simulink model "Combined_TorqueIncrease"  (Simulink 7.6)
settings: Solver=ode23tb  StartTime=0.0  StopTime=5  RelTol=1e-3
libraries: powerlib x14, powerlib_extras x1
settings Model: Creator=kif  LastModifiedBy=kif

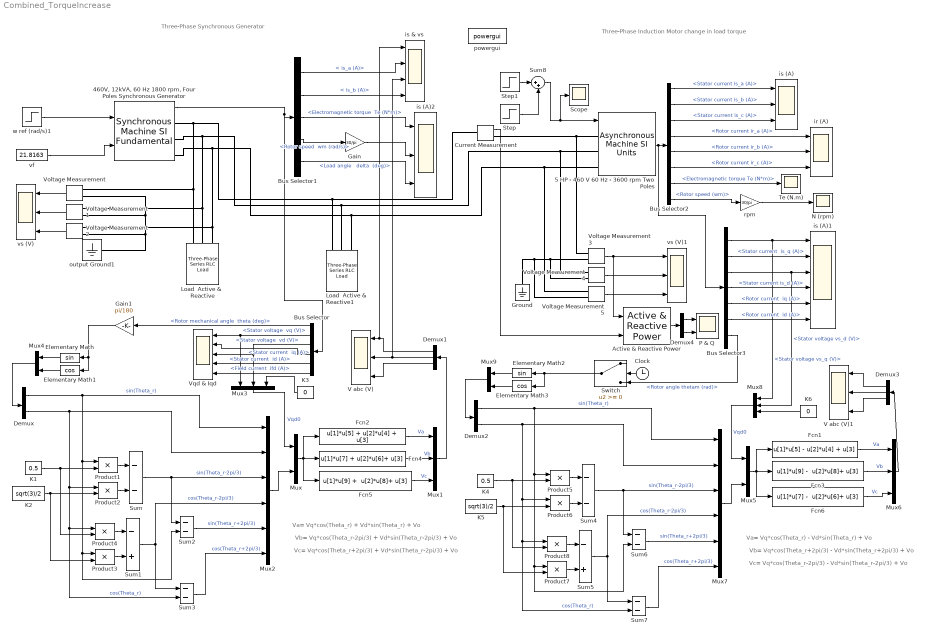
== system Combined_TorqueIncrease ==
  note: Three-Phase Synchronous Generator
  note: Va= Vq*cos(Theta_r) + Vd*sin(Theta_r) + Vo
  note: Vc= Vq*cos(Theta_r+2pi/3) + Vd*sin(Theta_r-2pi/3) + Vo
  note: Vb= Vq*cos(Theta_r-2pi/3) + Vd*sin(Theta_r-2pi/3) + Vo
  note: Three-Phase Induction Motor change in load torque
  note: Va= Vq*cos(Theta_r) - Vd*sin(Theta_r) + Vo
  note: Vc= Vq*cos(Theta_r-2pi/3) - Vd*sin(Theta_r-2pi/3) + Vo
  note: Vb= Vq*cos(Theta_r+2pi/3) - Vd*sin(Theta_r+2pi/3) + Vo
  "460V, 12kVA, 60 Hz 1800 rpm, Four Poles Synchronous Generator" : powerlib/Machines/Synchronous Machine SI Fundamental  DialogController=POWERSYS.PowerSysDialog  SystemSampleTime=-1  PresetModel=No  MechanicalLoad=Speed w  ShowDetailedParameters=on  RotorType=Salient-pole  NominalParameters="[ 11.9e3 460  60  0]"  Stator=[ .26 1.14e-3 13.7e-3 11.0e-3 ]  Field=[ 0.3 2.1e-3 ]  Dampers2=[ 1 2 3 4 5 6 ]  Dampers1=[ 0.0224 1.4e-3 0.02 1e-3 ]  Mechanical=[ 24.9 0 2]  PolePairs=2  InitialConditions=[0 -111.483 0 0 0 -173.297 66.7033 -53.2967 17.88]  SetSaturation=off  Saturation=[46.376,51.647,61.167,66.773,72.147,78.393,86.24,95.347,105.58;644,708.2,816.2,870.87,917.13,962.47,1012,1059.3,1104.5]  DisplayVfd=off  Units=SI fundamental parameters  LoadFlowParameters=[1 -50000 0 0 0]  TsPowergui=0  TsBlock=-1  IterativeModel=Forward Euler
      link override From: GotoTag=tp5344ed80_c545_43ed_8e4c_276f4009b387
      settings: AttributesFormatString=\n
  5 HP - 460 V 60 Hz - 3600 rpm Two Poles : powerlib/Machines/Asynchronous Machine SI Units  DialogController=POWERSYS.PowerSysDialog  SystemSampleTime=-1  PresetModel=No  MechanicalLoad=Torque Tm  ShowDetailedParameters=on  RotorType=Squirrel-cage  ReferenceFrame=Stationary  NominalParameters=[3730 460 60]  Stator=[1.115 0.005974]  Rotor=[1.083 0.005974]  Cage1=[ 0.022 0.226/377]  Cage2=[ 0.022 0.226/377]  Lm=0.2037  Mechanical=[0.02 0.005752 2]  PolePairs=2  InitialConditions="[ 1,0   0,0,0   0,0,0 ]"  Units=SI  LoadFlowParameters=0  SimulateSaturation=off  Saturation=[14.03593122, 27.81365428, 53.79336849, 72.68890987, 97.98006896, 148.6815601, 215.7428561, 302.9841135, 428.7778367 ; 230, 322, 414, 460, 506, 552, 598, 644, 690]  TsPowergui=0  TsBlock=-1  IterativeModel=Forward Euler
  Active & Reactive Power : powerlib_extras/Measurements/Active & Reactive Power  DialogController=POWERSYS.PowerSysDialog  SystemSampleTime=-1  f1=60
  Bus Selector : BusSelector  OutputSignals="Mechanical.Rotor mechanical angle  theta (deg),dq0 components.Stator voltage  vq (V),dq0 components.Stator voltage  vd (V),dq0 components.Stator current  iq (A),dq0 components.Stator current  id (A),dq0 components.Field current  ifd (A)"
  Bus Selector1 : BusSelector  OutputSignals="Stator current. is_a (A),Stator current. is_b (A),Mechanical.Electromagnetic torque  Te (N*m),Mechanical.Rotor speed  wm (rad/s),Load angle   delta  (deg)"
  Bus Selector2 : BusSelector  OutputSignals=Stator measurements.Stator current is_a (A),Stator measurements.Stator current is_b (A),Stator measurements.Stator current is_c (A),Rotor measurements.Rotor current ir_a (A),Rotor measurements.Rotor current ir_b (A),Rotor measurements.Rotor current ir_c (A),Mechanical.Electromagnetic torque Te (N*m),Mechanical.Rotor speed (wm)
  Bus Selector3 : BusSelector  OutputSignals="Stator measurements.Stator voltage vs_q (V),Stator measurements.Stator current  is_q (A),Stator measurements.Stator voltage vs_d (V),Stator measurements.Stator current is_d (A),Rotor measurements.Rotor current  iq (A),Rotor measurements.Rotor current  id (A),Mechanical.Rotor angle thetam (rad)"
  Clock : Clock
      settings: Decimation=10
  Current Measurement : powerlib/Measurements/Current Measurement  DialogController=POWERSYS.PowerSysDialog  SystemSampleTime=-1  PhasorSimulation=off  OutputType=Complex  PSBequivalent=0
  Demux : Demux  Outputs=2
  Demux1 : Demux  Outputs=3
  Demux2 : Demux  Outputs=2
  Demux3 : Demux  Outputs=3
  Demux4 : Demux  Outputs=2
  Elementary Math : Trigonometry
  Elementary Math1 : Trigonometry  Operator=cos
  Elementary Math2 : Trigonometry
  Elementary Math3 : Trigonometry  Operator=cos
  Fcn1 : Fcn  Expr="u[1]*u[5] -  u[2]*u[4] + u[3]"
  Fcn2 : Fcn  Expr=u[1]*u[5] + u[2]*u[4] + u[3]
  Fcn3 : Fcn  Expr="u[1]*u[9] -  u[2]*u[8]+ u[3]"
  Fcn4 : Fcn  Expr="u[1]*u[7] +  u[2]*u[6]+ u[3]"
  Fcn5 : Fcn  Expr="u[1]*u[9] +  u[2]*u[8]+ u[3]"
  Fcn6 : Fcn  Expr="u[1]*u[7] -  u[2]*u[6]+ u[3]"
  Gain : Gain  Gain=30/pi  SaturateOnIntegerOverflow=on  OutDataTypeStr=Inherit: Same as input  ParamDataTypeStr=Inherit: Same as input
  Gain1 : Gain  Gain=pi/180  SaturateOnIntegerOverflow=on  OutDataTypeStr=Inherit: Same as input  ParamDataTypeStr=Inherit: Same as input
  Ground : powerlib/Elements/Ground  DialogController=POWERSYS.PowerSysDialog  PhysicalDomain=powersysdomain  SubClassName=unknown  LeftPortType=p1  RightPortType=p1  LConnTagsString=a
  K1 : Constant  Value=0.5
  K2 : Constant  Value=sqrt(3)/2
  K3 : Constant  Value=0
  K4 : Constant  Value=0.5
  K5 : Constant  Value=sqrt(3)/2
  K6 : Constant  Value=0
  Load  Active &  Reactive : powerlib/Elements/Three-Phase Series RLC Load  DialogController=POWERSYS.PowerSysDialog  PhysicalDomain=powersysdomain  SubClassName=unknown  LeftPortType=p1  RightPortType=p1  LConnTagsString=A|B|C  Configuration=Y (grounded)  NominalVoltage=460  NominalFrequency=60  ActivePower=100  InductivePower=0  CapacitivePower=0  Measurements=None
  Load  Active &  Reactive1 : powerlib/Elements/Three-Phase Series RLC Load  DialogController=POWERSYS.PowerSysDialog  PhysicalDomain=powersysdomain  SubClassName=unknown  LeftPortType=p1  RightPortType=p1  LConnTagsString=A|B|C  Configuration=Y (grounded)  NominalVoltage=460  NominalFrequency=60  ActivePower=1000  InductivePower=100  CapacitivePower=0  Measurements=None
  Mux{,4..5,9} (4 alike) : Mux  Inputs=2
  Mux{1,3,6,8} (4 alike) : Mux  Inputs=3
  Mux2 : Mux  Inputs=6
  Mux7 : Mux  Inputs=6
  N (rpm) : Scope
      settings: TimeRange=1  YMin=0  YMax=4000  SaveName=ScopeData7  DataFormat=Structure
  P & Q : Scope  NumInputPorts=2
      settings: TimeRange=1  YMin=77.90000000000001~754  YMax=80.09999999999999~762.5  SaveName=ScopeData13  DataFormat=Structure
  Product{1..8} (8 alike) : Product  SaturateOnIntegerOverflow=on  InputSameDT=on  OutDataTypeStr=Inherit: Same as first input
  Scope : Scope
      settings: YMax=30  SaveName=ScopeData6
  Step : Step  Time=0  After=0  SampleTime=1
  Step1 : Step  Time=3  After=20  SampleTime=1
  Sum{,2..4,6..7} (6 alike) : Sum  Inputs=--  SaturateOnIntegerOverflow=on  InputSameDT=on  OutDataTypeStr=Inherit: Same as first input
  Sum1 : Sum  Inputs=-+  SaturateOnIntegerOverflow=on  InputSameDT=on  OutDataTypeStr=Inherit: Same as first input
  Sum5 : Sum  Inputs=-+  SaturateOnIntegerOverflow=on  InputSameDT=on  OutDataTypeStr=Inherit: Same as first input
  Sum8 : Sum  Inputs=|++
  Switch : Switch
  Te (N.m) : Scope
      settings: YMin=6  YMax=14  SaveName=ScopeData8  DataFormat=Structure
  V abc (V) : Scope  NumInputPorts=3
      settings: YMin=-3.5~-5~-5  YMax=3.5~5~5  DataFormat=Structure
  V abc (V)1 : Scope  NumInputPorts=3
      settings: YMin=-3.5~-5~-5  YMax=3.5~5~5  SaveName=ScopeData5  DataFormat=Structure
  Voltage Measurement{,1..5} (6 alike) : powerlib/Measurements/Voltage Measurement  DialogController=POWERSYS.PowerSysDialog  SystemSampleTime=-1  PhasorSimulation=off  OutputType=Complex  PSBequivalent=0
  Vqd & Iqd : Scope  NumInputPorts=5
      settings: YMin=-3.5~-5~-5~-5~-5  YMax=3.5~5~5~5~5  SaveName=ScopeData4  DataFormat=Structure
  ir (A) : Scope  NumInputPorts=3
      settings: YMin=-3.5~-5~-5  YMax=3.5~5~5  SaveName=ScopeData9  DataFormat=Structure
  is & vs : Scope  NumInputPorts=4
      settings: YMin=-300~-75~-300~-75  YMax=300~75~300~75  SaveName=ScopeData2  DataFormat=Structure
  is (A) : Scope  NumInputPorts=3
      settings: YMin=-8~-8~-8  YMax=8~8~8  SaveName=ScopeData10  DataFormat=Structure
  is (A)1 : Scope  NumInputPorts=6
      settings: YMin=-400~-7.5~-400~-7.5~-7.5~-7.5  YMax=400~7.5~400~7.5~7.5~7.5  SaveName=ScopeData11  DataFormat=Structure
  is (A)2 : Scope  NumInputPorts=3
      settings: TimeRange=3  YMin=53.875~1710~16.25  YMax=54.1~1890~16.725  SaveName=ScopeData3  DataFormat=Structure
  output Ground1 : powerlib/Elements/Ground  DialogController=POWERSYS.PowerSysDialog  PhysicalDomain=powersysdomain  SubClassName=unknown  LeftPortType=p1  RightPortType=p1  LConnTagsString=a
  powergui : powerlib/powergui  SystemSampleTime=-1  SimulationMode=Continuous  SampleTime=0  frequency=60  SPID=off  DisableSnubberDevices=off  DisableRonSwitches=off  DisableVfSwitches=off  SwTol=0  Interpol=off  frequencyindice=60  echomessages=off  HookPort=off  DisplayEquations=off  FunctionMessages=off  EnableUseOfTLC=off  x0status=blocks  RestoreLinks=warning  ResistiveCurrentMeasurement=off  Frange=[0:2:500]  Ylog=off  Xlog=on  ShowGrid=off  save=off  variable=ZData  ZoomFFT=off  StartTime=0.0  cycles=1  DisplayStyle=1  fundamental=60  FreqAxis=off  MaxFrequency=1000  frequencyindicesteady=1  RmsSteady=2  display=off  Ts=0  methode=off
  rpm : Gain  Gain=30/pi  SaturateOnIntegerOverflow=on  OutDataTypeStr=Inherit: Same as input  ParamDataTypeStr=Inherit: Same as input
  vf : Constant  Value=21.8163
  vs (V) : Scope  NumInputPorts=3
      settings: YMin=-3.5~-5~-5  YMax=3.5~5~5  DataFormat=Structure
  vs (V)1 : Scope  NumInputPorts=3
      settings: YMin=-300~-300~-300  YMax=300~300~300  SaveName=ScopeData12  DataFormat=Structure
  w ref (rad/s)1 : Step  Time=0  Before=188.4956  After=188.4956  SampleTime=0
  wires:
  vf/1 -> "460V, 12kVA, 60 Hz 1800 rpm, Four Poles Synchronous Generator"/2
  Voltage Measurement/1 -> vs (V)/1
  Voltage Measurement1/1 -> vs (V)/2
  Voltage Measurement2/1 -> vs (V)/3
  Fcn5/1 -> Mux1/3  "Vc"
  Fcn2/1 -> Mux1/1  "Va"
  Mux1/1 -> Demux1/1
  Mux/1 -> Fcn2/1, Fcn5/1, Fcn4/1
  Sum1/1 -> Sum3/1, Mux2/4  "cos(Theta_r-2pi/3)"
  Sum/1 -> Sum2/1, Mux2/3  "sin(Theta_r-2pi/3)"
  K2/1 -> Product3/2, Product2/2
  K1/1 -> Product4/2, Product1/2
  Sum2/1 -> Mux2/5  "sin(Theta_r+2pi/3)"
  Sum3/1 -> Mux2/6  "cos(Theta_r+2pi/3)"
  Product3/1 -> Sum1/2
  Product4/1 -> Sum1/1
  Product2/1 -> Sum/2
  Product1/1 -> Sum/1
  Demux/1 -> Mux2/1, Sum2/2, Product3/1, Product1/1  "sin(Theta_r)"
  Demux/2 -> Mux2/2, Product2/1, Product4/1, Sum3/2  "cos(Theta_r)"
  Mux4/1 -> Demux/1
  Mux2/1 -> Mux/2
  Mux3/1 -> Mux/1  "Vqd0"
  Elementary Math/1 -> Mux4/1
  Elementary Math1/1 -> Mux4/2
  Demux1/1 -> V abc (V)/1, is & vs/1
  Demux1/2 -> V abc (V)/2, is & vs/3
  Demux1/3 -> V abc (V)/3
  Bus Selector/2 -> Mux3/1, Vqd & Iqd/1  "<Stator voltage  vq (V)>"
  Bus Selector/3 -> Mux3/2, Vqd & Iqd/3  "<Stator voltage  vd (V)>"
  K3/1 -> Mux3/3
  Bus Selector/1 -> Gain1/1  "<Rotor mechanical angle  theta (deg)>"
  Fcn4/1 -> Mux1/2  "Vb"
  Bus Selector1/1 -> is & vs/2  "< is_a (A)>"
  Bus Selector1/2 -> is & vs/4  "< is_b (A)>"
  Bus Selector1/3 -> is (A)2/1  "<Electromagnetic torque  Te (N*m)>"
  Bus Selector1/4 -> Gain/1  "<Rotor speed  wm (rad/s)>"
  Bus Selector1/5 -> is (A)2/3  "<Load angle   delta  (deg)>"
  "460V, 12kVA, 60 Hz 1800 rpm, Four Poles Synchronous Generator"/1 -> Bus Selector1/1, Bus Selector/1
  Gain/1 -> is (A)2/2
  Gain1/1 -> Elementary Math/1, Elementary Math1/1
  w ref (rad/s)1/1 -> "460V, 12kVA, 60 Hz 1800 rpm, Four Poles Synchronous Generator"/1
  Bus Selector/5 -> Vqd & Iqd/4  "<Stator current  id (A)>"
  Bus Selector/4 -> Vqd & Iqd/2  "<Stator current  iq (A)>"
  Bus Selector/6 -> Vqd & Iqd/5  "<Field current  ifd (A)>"
  Bus Selector2/7 -> Te (N.m)/1  "<Electromagnetic torque Te (N*m)>"
  rpm/1 -> N (rpm)/1
  5 HP - 460 V 60 Hz - 3600 rpm Two Poles/1 -> Bus Selector2/1, Bus Selector3/1
  Bus Selector2/8 -> rpm/1  "<Rotor speed (wm)>"
  Bus Selector2/1 -> is (A)/1  "<Stator current is_a (A)>"
  Bus Selector2/2 -> is (A)/2  "<Stator current is_b (A)>"
  Bus Selector2/3 -> is (A)/3  "<Stator current is_c (A)>"
  Bus Selector2/4 -> ir (A)/1  "<Rotor current ir_a (A)>"
  Bus Selector2/5 -> ir (A)/2  "<Rotor current ir_b (A)>"
  Bus Selector2/6 -> ir (A)/3  "<Rotor current ir_c (A)>"
  Voltage Measurement3/1 -> vs (V)1/1, Active & Reactive Power/1
  Voltage Measurement4/1 -> vs (V)1/2
  Sum8/1 -> 5 HP - 460 V 60 Hz - 3600 rpm Two Poles/1, Scope/1
  Voltage Measurement5/1 -> vs (V)1/3
  Bus Selector3/1 -> is (A)1/1, Mux8/1  "<Stator voltage vs_q (V)>"
  Bus Selector3/2 -> is (A)1/2  "<Stator current  is_q (A)>"
  Bus Selector3/3 -> is (A)1/3, Mux8/2  "<Stator voltage vs_d (V)>"
  Bus Selector3/6 -> is (A)1/6  "<Rotor current  id (A)>"
  Bus Selector3/5 -> is (A)1/5  "<Rotor current  iq (A)>"
  Bus Selector3/4 -> is (A)1/4  "<Stator current is_d (A)>"
  Fcn6/1 -> Mux6/3  "Vc"
  Fcn1/1 -> Mux6/1  "Va"
  Mux6/1 -> Demux3/1
  Mux5/1 -> Fcn1/1, Fcn3/1, Fcn6/1
  Sum5/1 -> Sum7/1, Mux7/4  "cos(Theta_r-2pi/3)"
  Sum4/1 -> Sum6/1, Mux7/3  "sin(Theta_r-2pi/3)"
  K5/1 -> Product7/2, Product6/2
  K4/1 -> Product8/2, Product5/2
  Sum6/1 -> Mux7/5  "sin(Theta_r+2pi/3)"
  Sum7/1 -> Mux7/6  "cos(Theta_r+2pi/3)"
  Product7/1 -> Sum5/2
  Product8/1 -> Sum5/1
  Product6/1 -> Sum4/2
  Product5/1 -> Sum4/1
  Demux2/1 -> Mux7/1, Sum6/2, Product7/1, Product5/1  "sin(Theta_r)"
  Demux2/2 -> Mux7/2, Product6/1, Product8/1, Sum7/2  "cos(Theta_r)"
  Mux9/1 -> Demux2/1
  Mux7/1 -> Mux5/2
  Mux8/1 -> Mux5/1  "Vqd0"
  Fcn3/1 -> Mux6/2  "Vb"
  K6/1 -> Mux8/3
  Bus Selector3/7 -> Switch/3  "<Rotor angle thetam (rad)>"
  Elementary Math2/1 -> Mux9/1
  Elementary Math3/1 -> Mux9/2
  Switch/1 -> Elementary Math3/1, Elementary Math2/1
  Clock/1 -> Switch/2
  Demux3/2 -> V abc (V)1/2
  Demux3/3 -> V abc (V)1/3
  Step1/1 -> Sum8/1
  Step/1 -> Sum8/2
  Demux3/1 -> V abc (V)1/1
  Current Measurement/1 -> Active & Reactive Power/2
  Demux4/1 -> P & Q/1
  Demux4/2 -> P & Q/2
  Active & Reactive Power/1 -> Demux4/1
  connections:
  Current Measurement/RConn1 -- Voltage Measurement3/LConn1 -- 5 HP - 460 V 60 Hz - 3600 rpm Two Poles/LConn1
  5 HP - 460 V 60 Hz - 3600 rpm Two Poles/LConn2 -- Voltage Measurement4/LConn1 -- Load  Active &  Reactive/LConn2 -- Voltage Measurement1/LConn1 -- "460V, 12kVA, 60 Hz 1800 rpm, Four Poles Synchronous Generator"/RConn2 -- Load  Active &  Reactive1/LConn2
  5 HP - 460 V 60 Hz - 3600 rpm Two Poles/LConn3 -- Voltage Measurement5/LConn1 -- Load  Active &  Reactive/LConn3 -- Voltage Measurement2/LConn1 -- "460V, 12kVA, 60 Hz 1800 rpm, Four Poles Synchronous Generator"/RConn3 -- Load  Active &  Reactive1/LConn3
  output Ground1/LConn1 -- Voltage Measurement/LConn2 -- Voltage Measurement1/LConn2 -- Voltage Measurement2/LConn2
  Ground/LConn1 -- Voltage Measurement3/LConn2 -- Voltage Measurement4/LConn2 -- Voltage Measurement5/LConn2
  Load  Active &  Reactive/LConn1 -- Voltage Measurement/LConn1 -- "460V, 12kVA, 60 Hz 1800 rpm, Four Poles Synchronous Generator"/RConn1 -- Load  Active &  Reactive1/LConn1 -- Current Measurement/LConn1
